simulink model "JX_Kinect"  (Simulink 7.7)
settings: Solver=ode45  StartTime=0.0  StopTime=inf  FixedStep=sample_time  RelTol=1e-3
InitFcn:
  | sample_time=0.01;
undefined symbols (not defined in the file or in its folder): gray
libraries: vrlib x4, simulink_extras x3, nid_lib x2, vipsnks x1, utility x1
(part 1 of 2)
settings Model: Creator=ttcl3  LastModifiedBy=Jx
settings SolverCC: MaxConsecutiveMinStep=auto
settings DebuggingCC: MultiTaskRateTransMsg=warning

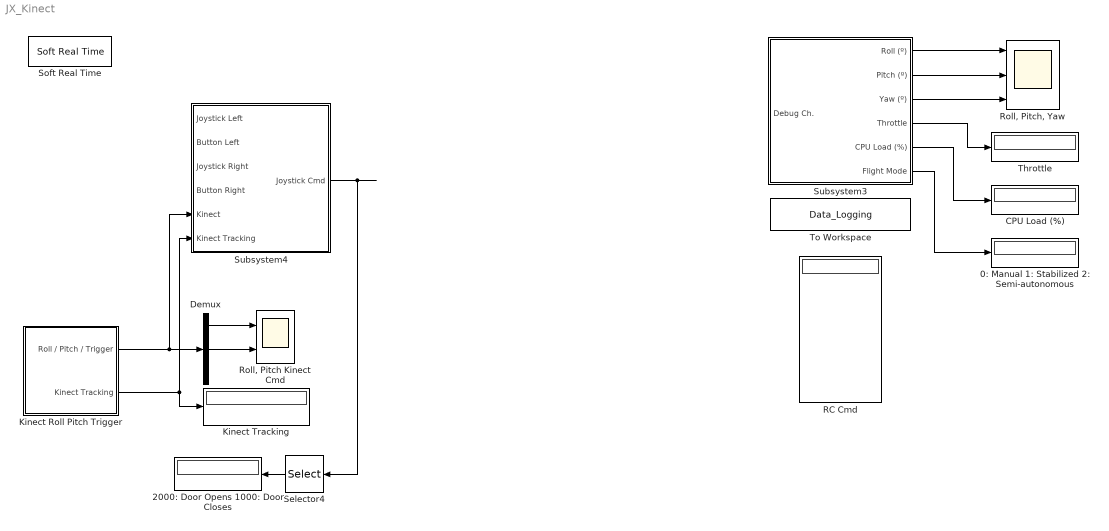
== system JX_Kinect ==
  0: Manual 1: Stabilized 2: Semi-autonomous : Display
  2000: Door Opens 1000: Door Closes : Display
  CPU Load (%) : Display
  Demux : Demux  Outputs=3
  Kinect Roll Pitch Trigger : Subsystem
      mask Display: image(imread('kinect.jpg'));port_label('output', 1, 'Roll/Pitch/Trigger'); port_label('output', 2, 'Tracking');
  Kinect Tracking : Display
  RC Cmd : Display
  "Roll, Pitch Kinect Cmd" : Scope  NumInputPorts=2
      settings: TickLabels=on  TimeRange=24  YMin=-90~-90  YMax=90~90  SampleInput=on
  "Roll, Pitch, Yaw" : Scope  NumInputPorts=3
      settings: TickLabels=on  TimeRange=24  YMin=-90~-90~-90  YMax=90~90~90  SampleInput=on
  Selector4 : Selector  InputPortWidth=7  IndexOptions=Index vector (dialog)  Indices=3  OutputSizes=1
  Soft Real Time : utility/Soft Real Time  x=0.8
  Subsystem3 : Subsystem
  Subsystem4 : Subsystem
  Throttle : Display
  To Workspace : ToWorkspace  VariableName=Data_Logging  SampleTime=-1  SaveFormat=Structure With Time
  wires:
  ? -> RC Cmd/1
  Subsystem3/1(Roll (º)) -> "Roll, Pitch, Yaw"/1
  Subsystem3/2(Pitch (º)) -> "Roll, Pitch, Yaw"/2
  Subsystem3/3(Yaw (º)) -> "Roll, Pitch, Yaw"/3
  Subsystem3/4(Throttle) -> Throttle/1
  Subsystem3/5(CPU Load (%)) -> CPU Load (%)/1
  Subsystem3/6(Flight Mode) -> 0: Manual 1: Stabilized 2: Semi-autonomous/1
  ? -> Subsystem3/1(Debug Ch.), To Workspace/1
  Subsystem4/1(Joystick Cmd) -> Selector4/1
  Kinect Roll Pitch Trigger/1(Roll / Pitch / Trigger) -> Subsystem4/5(Kinect), Demux/1
  Selector4/1 -> 2000: Door Opens 1000: Door Closes/1
  Kinect Roll Pitch Trigger/2(Kinect Tracking) -> Kinect Tracking/1, Subsystem4/6(Kinect Tracking)
  Demux/1 -> "Roll, Pitch Kinect Cmd"/1
  Demux/2 -> "Roll, Pitch Kinect Cmd"/2

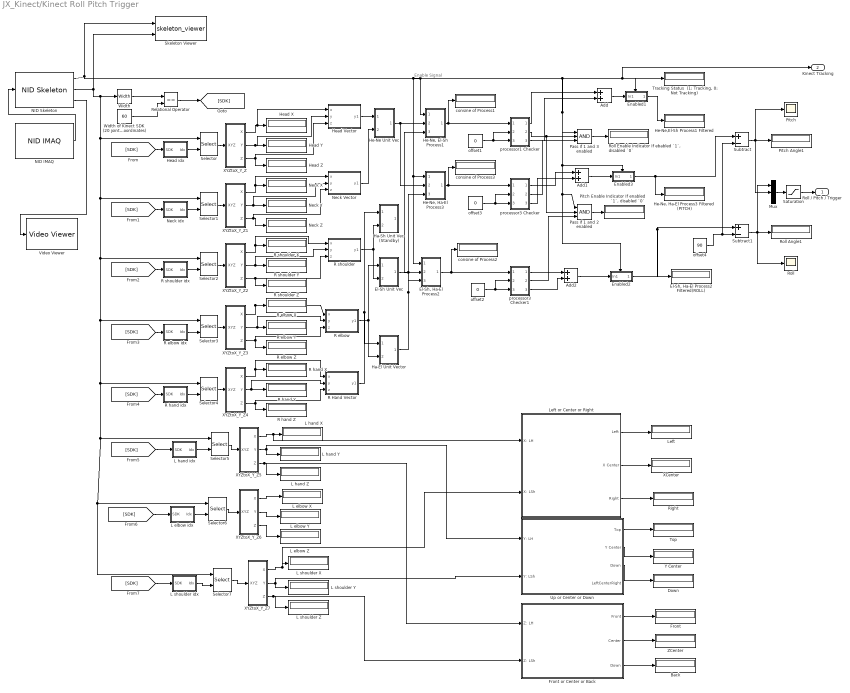
== system JX_Kinect/Kinect Roll Pitch Trigger ==
  note: Enable Signal
  Add : Sum
  Add1 : Sum
  Add2 : Sum
  Back : Display
  Down : Display
  El-Sh Unit Vec : Subsystem
  "El-Sh, Ha-El Process2" : Subsystem
  "El-Sh, Ha-El Process2 Filtered(ROLL)" : Display
  Enabled1 : Subsystem  TreatAsAtomicUnit=on
  Enabled2 : Subsystem  TreatAsAtomicUnit=on
  Enabled3 : Subsystem  TreatAsAtomicUnit=on
  Front : Display
  Front or Center or Back : Subsystem
  Ha-El Unit Vector : Subsystem
  Ha-Sh Unit Vec (Standby) : Subsystem
  He-Ne Unit Vec : Subsystem
  "He-Ne, El-Sh Process1" : Subsystem
  "He-Ne, Ha-El Process3" : Subsystem
  "He-Ne, Ha-El Process3 Filtered (PITCH)" : Display
  "He-Ne,El-Sh Process1 Filtered " : Display
  Head Vector : Stateflow chart  TreatAsAtomicUnit=on
  Head X : Display
  Head Y : Display
  Head Z : Display
  Head idx : Subsystem
  L elbow X : Display
  L elbow Y : Display
  L elbow Z : Display
  L elbow idx : Subsystem
  L hand X : Display
  L hand Y : Display
  L hand Z : Display
  L hand idx : Subsystem
  L shoulder X : Display
  L shoulder Y : Display
  L shoulder Z : Display
  L shoulder idx : Subsystem
  Left : Display
  Left or Center or Right : Subsystem
  Mux : Mux  Inputs=3
  NID IMAQ : nid_lib/NID IMAQ  imaq_depth=off  imaq_motion=off  imaq_image=off  view_point=off  imaq_skeleton=on  imaq_ir=off  mirror_image=off  imaq_sample_time=1/25  res_fps=VGA (640x480): 30 FPS  needPsiPose=off  angle_input=off  angle=0  angle_read=off  near_mode=off  seated_mode=off  skeleton_smooth=[1.0 0.5 0.5 0.05 0.04]  infer_skeleton=on
  NID Skeleton : nid_lib/NID Skeleton  num_of_skeleton_tracking=1  conv_XYZ_RW=on  viewer=on
  Neck Vector : Stateflow chart  TreatAsAtomicUnit=on
  Neck X : Display
  Neck Y : Display
  Neck Z : Display
  Neck idx : Subsystem
  Pass if 1 and 2 enabled : Logic  Inputs=3  AllPortsSameDT=off  OutDataTypeStr=boolean
  Pass if 1 and 3 enabled : Logic  Inputs=3  AllPortsSameDT=off  OutDataTypeStr=boolean
  Pitch : Scope
      settings: YMin=-90  YMax=90  SaveName=ScopeData3
  Pitch Angle1 : Display
  "Pitch Enable Indicator If enabled `1`, disabled `0` " : Display
  R Hand Vector : Stateflow chart  TreatAsAtomicUnit=on
  R elbow : Stateflow chart  TreatAsAtomicUnit=on
  R elbow X : Display
  R elbow Y : Display
  R elbow Z : Display
  R elbow idx : Subsystem
  R hand X : Display
  R hand Y : Display
  R hand Z : Display
  R hand idx : Subsystem
  R shoulder : Stateflow chart  TreatAsAtomicUnit=on
  R shoulder X : Display
  R shoulder Y : Display
  R shoulder Z : Display
  R shoulder idx : Subsystem
  Relational Operator : RelationalOperator  Operator===  OutDataTypeStr=boolean
  Right : Display
  Roll : Scope
      settings: YMin=-90  YMax=90  SaveName=ScopeData2
  Roll Angle1 : Display
  "Roll Enable Indicator If ebabled `1`, disabled `0`" : Display
  Saturation : Saturate  UpperLimit=30  LowerLimit=-30
  Selector{,1..7} (8 alike) : Selector  NumberOfDimensions=3  InputPortWidth=3  IndexOptions=Select all,Index vector (port),Select all  Indices=[1 3],1,1  OutputSizes=1,1,1
  Skeleton Viewer : M-S-Function  FunctionName=skeleton_viewer
      mask Display:
      | disp('Skeleton\nViewer')
      | 
      | port_label('input', 1, 'Tracking')
      | port_label('input', 2, 'Skeleton')
  Subtract : Sum  Inputs=+-
  Subtract1 : Sum  Inputs=+-
  Top : Display
  "Tracking Status  (1: Tracking, 0: Not Tracking)" : Display
  Up or Center or Down : Subsystem
  Video Viewer : vipsnks/Video Viewer  inputType=Obsolete7b  imagePorts=One multidimensional signal  useColorMap=off  colormapValue=gray(256)  specRange=off  minInputVal=0  maxInputVal=255  FigPos=[1181 519 698 403]  AxisZoom=on  trueSizedOnce=off  OpenAtMdlStart=on
  Width : Width
  Width of Kinect SDK  (20 joints x 3 coordinates) : Constant  Value=60
  XCenter : Display
  XYZtoX_Y_Z : Subsystem
  XYZtoX_Y_Z1 : Subsystem
  XYZtoX_Y_Z2 : Subsystem
  XYZtoX_Y_Z3 : Subsystem
  XYZtoX_Y_Z4 : Subsystem
  XYZtoX_Y_Z5 : Subsystem
  XYZtoX_Y_Z6 : Subsystem
  XYZtoX_Y_Z7 : Subsystem
  Y Center : Display
  ZCenter : Display
  consine of Process1 : Display
  consine of Process2 : Display
  consine of Process3 : Display
  offset1 : Constant  Value=0
  offset2 : Constant  Value=0
  offset3 : Constant  Value=0
  offset4 : Constant  Value=90
  processor1 Checker : Subsystem
  processor3 Checker : Subsystem
  processor3 Checker1 : Subsystem
  Roll / Pitch / Trigger : Outport
  Kinect Tracking : Outport  Port=2
  wires:
  Saturation/1 -> Roll / Pitch / Trigger/1
  Mux/1 -> Saturation/1
  Pass if 1 and 3 enabled/1 -> "Roll Enable Indicator If ebabled `1`, disabled `0`"/1
  Subtract1/1 -> Roll/1, Mux/1, Roll Angle1/1
  Subtract/1 -> Pitch/1, Mux/2, Pitch Angle1/1
  offset4/1 -> Subtract/2, Subtract1/2
  Add2/1 -> Enabled2/1(In1)
  processor3 Checker1/3(Out3) -> Add2/2
  processor3 Checker1/1(Out1) -> Add2/1
  processor3 Checker/3(Out3) -> Add1/2
  processor3 Checker/1(Out1) -> Add1/1
  Add1/1 -> Enabled3/1(In1)
  processor1 Checker/1(Out1) -> Add/1
  Add/1 -> Enabled1/1(In1)
  processor1 Checker/3(Out3) -> Add/2
  Enabled2/1(Out1) -> Subtract1/1, "El-Sh, Ha-El Process2 Filtered(ROLL)"/1
  Enabled1/1(Out1) -> "He-Ne,El-Sh Process1 Filtered "/1
  Enabled3/1(Out1) -> Subtract/1, "He-Ne, Ha-El Process3 Filtered (PITCH)"/1
  offset2/1 -> processor3 Checker1/2(In2), processor3 Checker1/3(In3)
  offset3/1 -> processor3 Checker/2(In2), processor3 Checker/3(In3)
  offset1/1 -> processor1 Checker/2(In2), processor1 Checker/3(In3)
  processor3 Checker1/2(Out2) -> Pass if 1 and 2 enabled/3
  processor1 Checker/2(Out2) -> Pass if 1 and 2 enabled/2, Pass if 1 and 3 enabled/2
  processor3 Checker/2(Out2) -> Pass if 1 and 3 enabled/3
  Pass if 1 and 2 enabled/1 -> "Pitch Enable Indicator If enabled `1`, disabled `0` "/1
  "El-Sh, Ha-El Process2"/1(Out1) -> processor3 Checker1/1(In1), consine of Process2/1
  "He-Ne, El-Sh Process1"/1(Out1) -> consine of Process1/1, processor1 Checker/1(In1)
  "He-Ne, Ha-El Process3"/1(Out1) -> processor3 Checker/1(In1), consine of Process3/1
  Ha-El Unit Vector/1(Out1) -> "He-Ne, Ha-El Process3"/3(In3), "El-Sh, Ha-El Process2"/3(In3)
  El-Sh Unit Vec/1(Out1) -> "El-Sh, Ha-El Process2"/2(In2), "He-Ne, El-Sh Process1"/3(In3)
  He-Ne Unit Vec/1(Out1) -> "He-Ne, El-Sh Process1"/2(In2), "He-Ne, Ha-El Process3"/2(In2)
  R elbow/1(y1) -> Ha-El Unit Vector/2(In2), El-Sh Unit Vec/1(In1)
  R Hand Vector/1(y1) -> Ha-El Unit Vector/1(In1), Ha-Sh Unit Vec (Standby)/1(In1)
  R shoulder/1(y1) -> El-Sh Unit Vec/2(In2), Ha-Sh Unit Vec (Standby)/2(In2)
  Head Vector/1(y1) -> He-Ne Unit Vec/1(In1)
  Neck Vector/1(y1) -> He-Ne Unit Vec/2(In2)
  Selector/1 -> XYZtoX_Y_Z/1(XYZ)
  Selector4/1 -> XYZtoX_Y_Z4/1(XYZ)
  XYZtoX_Y_Z4/3(Z) -> R Hand Vector/3(z), R hand Z/1
  XYZtoX_Y_Z4/2(Y) -> R Hand Vector/2(y), R hand Y/1
  XYZtoX_Y_Z4/1(X) -> R Hand Vector/1(x), R hand X/1
  Selector3/1 -> XYZtoX_Y_Z3/1(XYZ)
  XYZtoX_Y_Z3/3(Z) -> R elbow/3(z), R elbow Z/1
  XYZtoX_Y_Z3/2(Y) -> R elbow/2(y), R elbow Y/1
  XYZtoX_Y_Z3/1(X) -> R elbow/1(x), R elbow X/1
  Selector2/1 -> XYZtoX_Y_Z2/1(XYZ)
  XYZtoX_Y_Z2/3(Z) -> R shoulder/3(z), R shoulder Z/1
  XYZtoX_Y_Z2/2(Y) -> R shoulder/2(y), R shoulder Y/1
  XYZtoX_Y_Z2/1(X) -> R shoulder/1(x), R shoulder X/1
  XYZtoX_Y_Z1/3(Z) -> Neck Vector/3(z), Neck Z/1
  XYZtoX_Y_Z1/2(Y) -> Neck Vector/2(y), Neck Y/1
  XYZtoX_Y_Z1/1(X) -> Neck Vector/1(x), Neck X/1
  XYZtoX_Y_Z/3(Z) -> Head Vector/3(z), Head Z/1
  XYZtoX_Y_Z/2(Y) -> Head Vector/2(y), Head Y/1
  [SDK] -> R hand idx/1(SDK)
  R hand idx/1(Idx) -> Selector4/2
  [SDK] -> R elbow idx/1(SDK)
  R elbow idx/1(Idx) -> Selector3/2
  [SDK] -> R shoulder idx/1(SDK)
  R shoulder idx/1(Idx) -> Selector2/2
  Selector1/1 -> XYZtoX_Y_Z1/1(XYZ)
  [SDK] -> Neck idx/1(SDK)
  Neck idx/1(Idx) -> Selector1/2
  XYZtoX_Y_Z/1(X) -> Head Vector/1(x), Head X/1
  NID Skeleton/1 -> "He-Ne, El-Sh Process1"/1(In1), Pass if 1 and 3 enabled/1, Kinect Tracking/1, "Tracking Status  (1: Tracking, 0: Not Tracking)"/1, Enabled1/Enable, Enabled3/Enable, Enabled2/Enable, Pass if 1 and 2 enabled/1, "He-Ne, Ha-El Process3"/1(In1), "El-Sh, Ha-El Process2"/1(In1), Skeleton Viewer/1
  [SDK] -> Head idx/1(SDK)
  Head idx/1(Idx) -> Selector/2
  Relational Operator/1 -> [SDK]
  NID Skeleton/2 -> Selector3/1, Selector4/1, Selector5/1, Selector6/1, Selector7/1, Selector2/1, Selector1/1, Selector/1, Width/1, Skeleton Viewer/2
  Width of Kinect SDK  (20 joints x 3 coordinates)/1 -> Relational Operator/2
  Width/1 -> Relational Operator/1
  NID IMAQ/1 -> NID Skeleton/1
  [SDK] -> L hand idx/1(SDK)
  [SDK] -> L elbow idx/1(SDK)
  [SDK] -> L shoulder idx/1(SDK)
  L hand idx/1(Idx) -> Selector5/2
  L elbow idx/1(Idx) -> Selector6/2
  L shoulder idx/1(Idx) -> Selector7/2
  Selector5/1 -> XYZtoX_Y_Z5/1(XYZ)
  XYZtoX_Y_Z5/1(X) -> L hand X/1, Left or Center or Right/1(X: LH)
  XYZtoX_Y_Z5/2(Y) -> L hand Y/1, Up or Center or Down/1(Y: LH)
  XYZtoX_Y_Z5/3(Z) -> L hand Z/1, Front or Center or Back/1(Z: LH)
  XYZtoX_Y_Z6/1(X) -> L elbow X/1
  XYZtoX_Y_Z6/2(Y) -> L elbow Y/1
  XYZtoX_Y_Z6/3(Z) -> L elbow Z/1
  XYZtoX_Y_Z7/1(X) -> L shoulder X/1, Left or Center or Right/2(X: LSh)
  XYZtoX_Y_Z7/2(Y) -> L shoulder Y/1, Up or Center or Down/2(Y: LSh)
  XYZtoX_Y_Z7/3(Z) -> L shoulder Z/1, Front or Center or Back/2(Z: LSh)
  Selector6/1 -> XYZtoX_Y_Z6/1(XYZ)
  Selector7/1 -> XYZtoX_Y_Z7/1(XYZ)
  Left or Center or Right/1(Left) -> Left/1
  Left or Center or Right/3(Right) -> Right/1
  Up or Center or Down/1(Top) -> Top/1
  Up or Center or Down/2(Y Center) -> Y Center/1
  Up or Center or Down/3(Down) -> Down/1
  Front or Center or Back/1(Front) -> Front/1
  Front or Center or Back/2(Center) -> ZCenter/1
  Front or Center or Back/3(Down) -> Back/1
  Left or Center or Right/2(X Center) -> XCenter/1
  NID Skeleton/3 -> Video Viewer/1

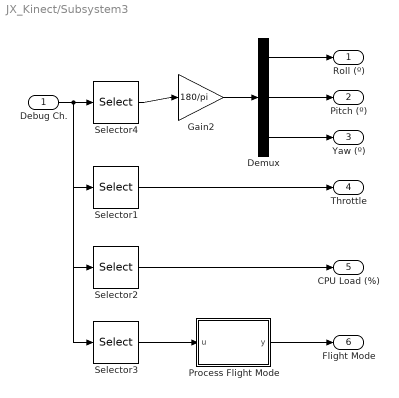
== system JX_Kinect/Subsystem3 ==
  Debug Ch. : Inport
  Demux : Demux  Outputs=3
  Gain2 : Gain  Gain=180/pi
  Process Flight Mode : Stateflow chart  TreatAsAtomicUnit=on
  Selector1 : Selector  InputPortWidth=6  IndexOptions=Index vector (dialog)  Indices=4  OutputSizes=1
  Selector2 : Selector  InputPortWidth=6  IndexOptions=Index vector (dialog)  Indices=5  OutputSizes=1
  Selector3 : Selector  InputPortWidth=6  IndexOptions=Index vector (dialog)  Indices=6  OutputSizes=1
  Selector4 : Selector  InputPortWidth=6  IndexOptions=Index vector (dialog)  Indices=[1 2 3]  OutputSizes=1
  Roll (º) : Outport
  Pitch (º) : Outport  Port=2
  Yaw (º) : Outport  Port=3
  Throttle : Outport  Port=4
  CPU Load (%) : Outport  Port=5
  Flight Mode : Outport  Port=6
  wires:
  Selector4/1 -> Gain2/1
  Gain2/1 -> Demux/1
  Demux/1 -> Roll (º)/1
  Demux/2 -> Pitch (º)/1
  Debug Ch./1 -> Selector4/1, Selector1/1, Selector2/1, Selector3/1
  Demux/3 -> Yaw (º)/1
  Selector1/1 -> Throttle/1
  Selector2/1 -> CPU Load (%)/1
  Selector3/1 -> Process Flight Mode/1(u)
  Process Flight Mode/1(y) -> Flight Mode/1

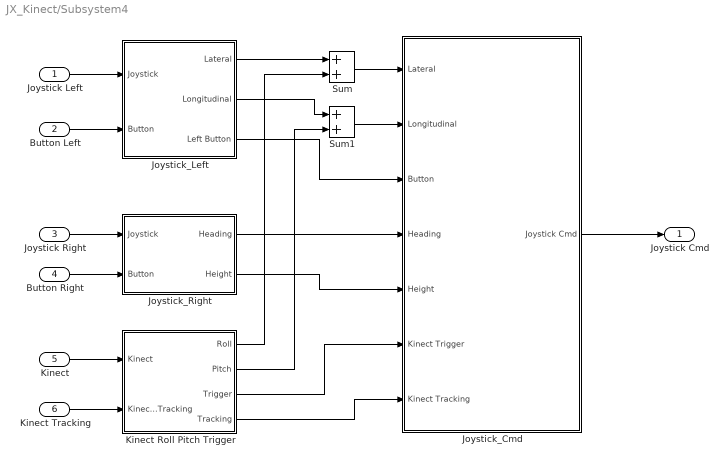
== system JX_Kinect/Subsystem4 ==
  Joystick Left : Inport
  Button Left : Inport  Port=2
  Joystick Right : Inport  Port=3
  Button Right : Inport  Port=4
  Kinect : Inport  Port=5
  Kinect Tracking : Inport  Port=6
  Joystick_Cmd : Subsystem
  Joystick_Left : Subsystem
  Joystick_Right : Subsystem
  Kinect Roll Pitch Trigger : Subsystem
  Sum : Sum
  Sum1 : Sum
  Joystick Cmd : Outport
  wires:
  Joystick Left/1 -> Joystick_Left/1(Joystick)
  Joystick Right/1 -> Joystick_Right/1(Joystick)
  Button Right/1 -> Joystick_Right/2(Button)
  Button Left/1 -> Joystick_Left/2(Button)
  Joystick_Right/1(Heading) -> Joystick_Cmd/4(Heading)
  Joystick_Right/2(Height) -> Joystick_Cmd/5(Height)
  Kinect/1 -> Kinect Roll Pitch Trigger/1(Kinect)
  Joystick_Left/3(Left Button) -> Joystick_Cmd/3(Button)
  Joystick_Cmd/1(Joystick Cmd) -> Joystick Cmd/1
  Joystick_Left/1(Lateral) -> Sum/1
  Sum/1 -> Joystick_Cmd/1(Lateral)
  Sum1/1 -> Joystick_Cmd/2(Longitudinal)
  Joystick_Left/2(Longitudinal) -> Sum1/1
  Kinect Roll Pitch Trigger/3(Trigger) -> Joystick_Cmd/6(Kinect Trigger)
  Kinect Tracking/1 -> Kinect Roll Pitch Trigger/2(Kinect Tracking)
  Kinect Roll Pitch Trigger/4(Tracking) -> Joystick_Cmd/7(Kinect Tracking)
  Kinect Roll Pitch Trigger/1(Roll) -> Sum/2
  Kinect Roll Pitch Trigger/2(Pitch) -> Sum1/2

== system JX_Kinect/Kinect Roll Pitch Trigger/El-Sh Unit Vec ==
  In1 : Inport
  In2 : Inport  Port=2
  Shoudler Elbow : vrlib/Utilities/Normalize Vector  SystemSampleTime=-1  maxzero=0
  Subtract3 : Sum  Inputs=+-
  Out1 : Outport
  wires:
  Shoudler Elbow/1 -> Out1/1
  In2/1 -> Subtract3/2
  In1/1 -> Subtract3/1
  Subtract3/1 -> Shoudler Elbow/1

== system JX_Kinect/Kinect Roll Pitch Trigger/El-Sh, Ha-El Process2 ==
  In1 : Inport
  In2 : Inport  Port=2
  In3 : Inport  Port=3
  Enabled Subsystem2 : Subsystem  TreatAsAtomicUnit=on
  "consine El-Sh, Ha-El" : DotProduct  InputSameDT=on  OutDataTypeStr=Inherit: Inherit via internal rule
  Out1 : Outport
  wires:
  Enabled Subsystem2/1(Out1) -> Out1/1
  In3/1 -> "consine El-Sh, Ha-El"/2
  In2/1 -> "consine El-Sh, Ha-El"/1
  In1/1 -> Enabled Subsystem2/Enable
  "consine El-Sh, Ha-El"/1 -> Enabled Subsystem2/1(In1)

== system JX_Kinect/Kinect Roll Pitch Trigger/Enabled1 ==
  In1 : Inport
  Enable : EnablePort
  Out1 : Outport
  wires:
  In1/1 -> Out1/1

== system JX_Kinect/Kinect Roll Pitch Trigger/Enabled2 ==
  In1 : Inport
  Enable : EnablePort
  Out1 : Outport
  wires:
  In1/1 -> Out1/1

== system JX_Kinect/Kinect Roll Pitch Trigger/Enabled3 ==
  In1 : Inport
  Enable : EnablePort
  Out1 : Outport
  wires:
  In1/1 -> Out1/1

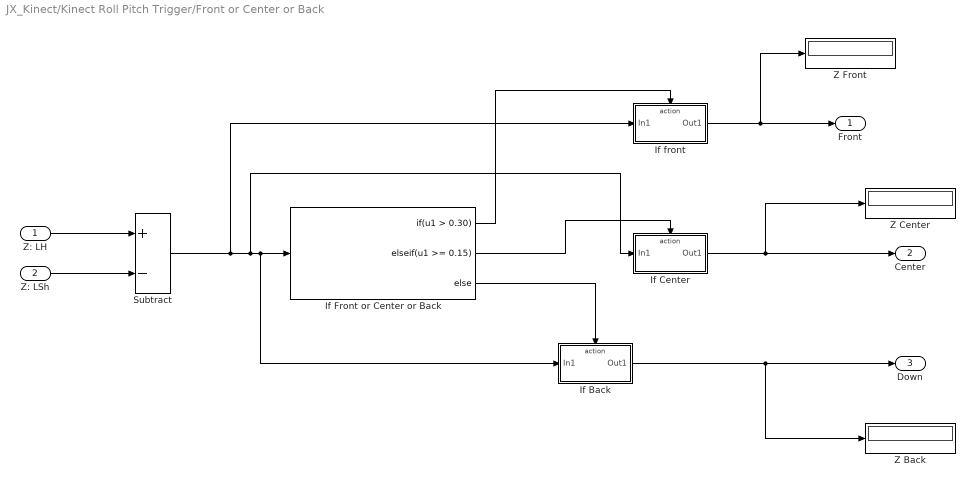
== system JX_Kinect/Kinect Roll Pitch Trigger/Front or Center or Back ==
  Z: LH : Inport
  Z: LSh : Inport  Port=2
  If Back : Subsystem  TreatAsAtomicUnit=on
  If Center : Subsystem  TreatAsAtomicUnit=on
  If Front or Center or Back : If  IfExpression=u1 > 0.30  ElseIfExpressions=u1 >= 0.15
  If front : Subsystem  TreatAsAtomicUnit=on
  Subtract : Sum  Inputs=+-
  Z Back : Display
  Z Center : Display
  Z Front : Display
  Front : Outport
  Center : Outport  Port=2
  Down : Outport  Port=3
  wires:
  Z: LH/1 -> Subtract/1
  Z: LSh/1 -> Subtract/2
  Subtract/1 -> If front/1(In1), If Center/1(In1), If Front or Center or Back/1, If Back/1(In1)
  If Front or Center or Back/1 -> If front/Action
  If front/1(Out1) -> Front/1, Z Front/1
  If Front or Center or Back/2 -> If Center/Action
  If Center/1(Out1) -> Center/1, Z Center/1
  If Front or Center or Back/3 -> If Back/Action
  If Back/1(Out1) -> Down/1, Z Back/1

== system JX_Kinect/Kinect Roll Pitch Trigger/Ha-El Unit Vector ==
  In1 : Inport
  In2 : Inport  Port=2
  Elbow Hand : vrlib/Utilities/Normalize Vector  SystemSampleTime=-1  maxzero=0
  Subtract2 : Sum  Inputs=+-
  Out1 : Outport
  wires:
  Elbow Hand/1 -> Out1/1
  In2/1 -> Subtract2/2
  In1/1 -> Subtract2/1
  Subtract2/1 -> Elbow Hand/1

== system JX_Kinect/Kinect Roll Pitch Trigger/Ha-Sh Unit Vec (Standby) ==
  In1 : Inport
  In2 : Inport  Port=2
  Subtract1 : Sum  Inputs=+-
  Unit Vector1 : vrlib/Utilities/Normalize Vector  SystemSampleTime=-1  maxzero=0
  Out1 : Outport
  wires:
  Unit Vector1/1 -> Out1/1
  In2/1 -> Subtract1/2
  In1/1 -> Subtract1/1
  Subtract1/1 -> Unit Vector1/1

== system JX_Kinect/Kinect Roll Pitch Trigger/He-Ne Unit Vec ==
  In1 : Inport
  In2 : Inport  Port=2
  Subtract : Sum  Inputs=+-
  Unit Vector : vrlib/Utilities/Normalize Vector  SystemSampleTime=-1  maxzero=0
  Out1 : Outport
  wires:
  In2/1 -> Subtract/2
  Unit Vector/1 -> Out1/1
  In1/1 -> Subtract/1
  Subtract/1 -> Unit Vector/1

== system JX_Kinect/Kinect Roll Pitch Trigger/He-Ne, El-Sh Process1 ==
  In1 : Inport
  In2 : Inport  Port=2
  In3 : Inport  Port=3
  Enabled Subsystem1 : Subsystem  TreatAsAtomicUnit=on
  consine He-Ne El-Sh : DotProduct  InputSameDT=on  OutDataTypeStr=Inherit: Inherit via internal rule
  Out1 : Outport
  wires:
  Enabled Subsystem1/1(Out1) -> Out1/1
  In3/1 -> consine He-Ne El-Sh/2
  In2/1 -> consine He-Ne El-Sh/1
  In1/1 -> Enabled Subsystem1/Enable
  consine He-Ne El-Sh/1 -> Enabled Subsystem1/1(In1)

== system JX_Kinect/Kinect Roll Pitch Trigger/He-Ne, Ha-El Process3 ==
  In1 : Inport
  In2 : Inport  Port=2
  In3 : Inport  Port=3
  Enabled Subsystem3 : Subsystem  TreatAsAtomicUnit=on
  "consine He-Ne, Ha-El" : DotProduct  InputSameDT=on  OutDataTypeStr=Inherit: Inherit via internal rule
  Out1 : Outport
  wires:
  Enabled Subsystem3/1(Out1) -> Out1/1
  In3/1 -> "consine He-Ne, Ha-El"/2
  In2/1 -> "consine He-Ne, Ha-El"/1
  In1/1 -> Enabled Subsystem3/Enable
  "consine He-Ne, Ha-El"/1 -> Enabled Subsystem3/1(In1)

== system JX_Kinect/Kinect Roll Pitch Trigger/Head idx ==
  SDK : Inport
  Kinect SDK : Constant  Value=4
  OpenNI : Constant
  Switch : Switch  Criteria=u2 ~= 0
  Idx : Outport
  wires:
  Switch/1 -> Idx/1
  SDK/1 -> Switch/2
  OpenNI/1 -> Switch/3
  Kinect SDK/1 -> Switch/1

== system JX_Kinect/Kinect Roll Pitch Trigger/L elbow idx ==
  SDK : Inport
  Kinect SDK : Constant  Value=6
  OpenNI : Constant  Value=8
  Switch : Switch  Criteria=u2 ~= 0
  Idx : Outport
  wires:
  Kinect SDK/1 -> Switch/1
  OpenNI/1 -> Switch/3
  SDK/1 -> Switch/2
  Switch/1 -> Idx/1

== system JX_Kinect/Kinect Roll Pitch Trigger/L hand idx ==
  SDK : Inport
  Kinect SDK : Constant  Value=8
  OpenNI : Constant  Value=9
  Switch : Switch  Criteria=u2 ~= 0
  Idx : Outport
  wires:
  Kinect SDK/1 -> Switch/1
  OpenNI/1 -> Switch/3
  SDK/1 -> Switch/2
  Switch/1 -> Idx/1

== system JX_Kinect/Kinect Roll Pitch Trigger/L shoulder idx ==
  SDK : Inport
  Kinect SDK : Constant  Value=5
  OpenNI : Constant  Value=7
  Switch : Switch  Criteria=u2 ~= 0
  Idx : Outport
  wires:
  Kinect SDK/1 -> Switch/1
  OpenNI/1 -> Switch/3
  SDK/1 -> Switch/2
  Switch/1 -> Idx/1

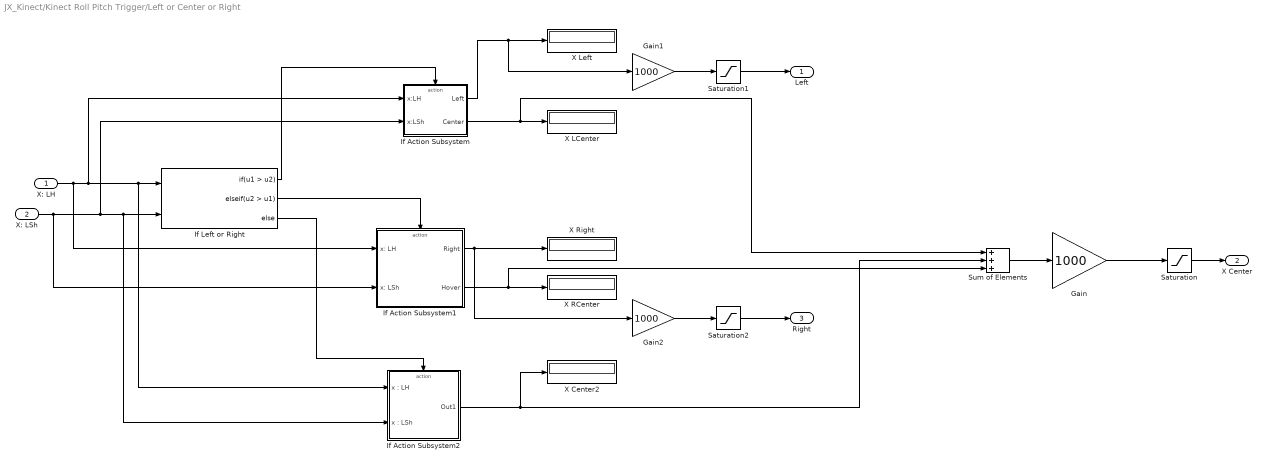
== system JX_Kinect/Kinect Roll Pitch Trigger/Left or Center or Right ==
  X: LH : Inport
  X: LSh : Inport  Port=2
  Gain : Gain  Gain=1000
  Gain1 : Gain  Gain=1000
  Gain2 : Gain  Gain=1000
  If Action Subsystem : Subsystem  TreatAsAtomicUnit=on
  If Action Subsystem1 : Subsystem  TreatAsAtomicUnit=on
  If Action Subsystem2 : Subsystem  TreatAsAtomicUnit=on
  If Left or Right : If  NumInputs=2  IfExpression=u1 > u2  ElseIfExpressions=u2 > u1
  Saturation : Saturate  UpperLimit=1  LowerLimit=0
  Saturation1 : Saturate  UpperLimit=1  LowerLimit=0
  Saturation2 : Saturate  UpperLimit=1  LowerLimit=0
  Sum of Elements : Sum  Inputs=+|+|+
  X Center2 : Display
  X LCenter : Display
  X Left : Display
  X RCenter : Display
  X Right : Display
  Left : Outport
  X Center : Outport  Port=2
  Right : Outport  Port=3
  wires:
  If Action Subsystem1/2(Hover) -> X RCenter/1, Sum of Elements/3
  If Action Subsystem1/1(Right) -> X Right/1, Gain2/1
  If Action Subsystem/2(Center) -> X LCenter/1, Sum of Elements/1
  If Left or Right/2 -> If Action Subsystem1/Action
  If Action Subsystem/1(Left) -> X Left/1, Gain1/1
  If Left or Right/1 -> If Action Subsystem/Action
  X: LH/1 -> If Action Subsystem/1(x:LH), If Left or Right/1, If Action Subsystem2/1("x : LH"), If Action Subsystem1/1(x: LH)
  X: LSh/1 -> If Action Subsystem/2(x:LSh), If Left or Right/2, If Action Subsystem2/2("x : LSh"), If Action Subsystem1/2(x: LSh)
  If Left or Right/3 -> If Action Subsystem2/Action
  If Action Subsystem2/1(Out1) -> X Center2/1, Sum of Elements/2
  Sum of Elements/1 -> Gain/1
  Gain/1 -> Saturation/1
  Saturation/1 -> X Center/1
  Gain1/1 -> Saturation1/1
  Saturation1/1 -> Left/1
  Gain2/1 -> Saturation2/1
  Saturation2/1 -> Right/1

== system JX_Kinect/Kinect Roll Pitch Trigger/Neck idx ==
  SDK : Inport
  Kinect SDK : Constant  Value=3
  OpenNI : Constant  Value=2
  Switch : Switch  Criteria=u2 ~= 0
  Idx : Outport
  wires:
  Kinect SDK/1 -> Switch/1
  OpenNI/1 -> Switch/3
  SDK/1 -> Switch/2
  Switch/1 -> Idx/1

== system JX_Kinect/Kinect Roll Pitch Trigger/R elbow idx ==
  SDK : Inport
  Kinect SDK : Constant  Value=10
  OpenNI : Constant  Value=5
  Switch : Switch  Criteria=u2 ~= 0
  Idx : Outport
  wires:
  Switch/1 -> Idx/1
  SDK/1 -> Switch/2
  OpenNI/1 -> Switch/3
  Kinect SDK/1 -> Switch/1

== system JX_Kinect/Kinect Roll Pitch Trigger/R hand idx ==
  SDK : Inport
  Kinect SDK : Constant  Value=12
  OpenNI : Constant  Value=6
  Switch : Switch  Criteria=u2 ~= 0
  Idx : Outport
  wires:
  Switch/1 -> Idx/1
  SDK/1 -> Switch/2
  OpenNI/1 -> Switch/3
  Kinect SDK/1 -> Switch/1

== system JX_Kinect/Kinect Roll Pitch Trigger/R shoulder idx ==
  SDK : Inport
  Kinect SDK : Constant  Value=9
  OpenNI : Constant  Value=4
  Switch : Switch  Criteria=u2 ~= 0
  Idx : Outport
  wires:
  Switch/1 -> Idx/1
  SDK/1 -> Switch/2
  OpenNI/1 -> Switch/3
  Kinect SDK/1 -> Switch/1

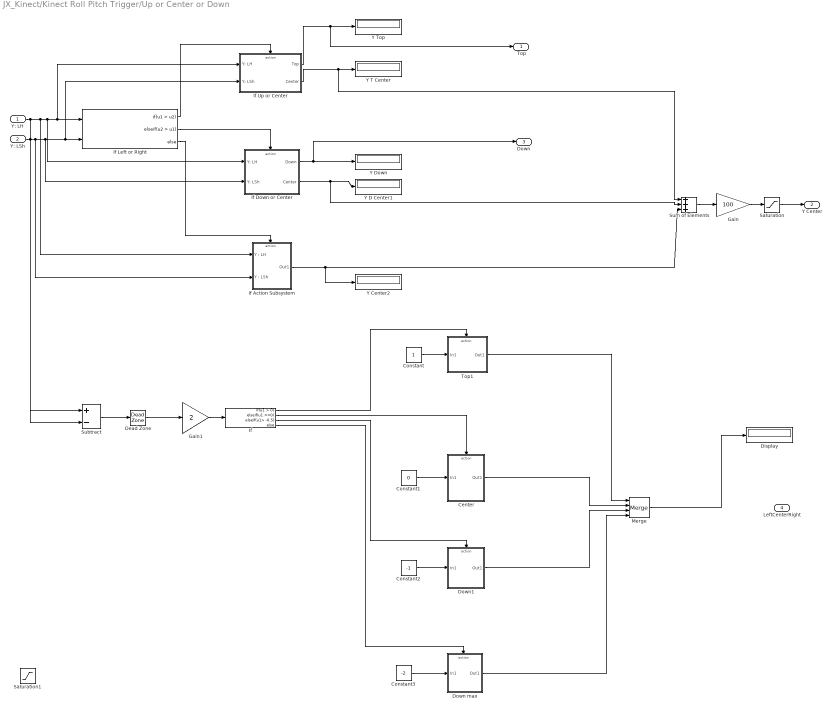
== system JX_Kinect/Kinect Roll Pitch Trigger/Up or Center or Down ==
  Y: LH : Inport
  Y: LSh : Inport  Port=2
  Center : Subsystem  TreatAsAtomicUnit=on
  Constant : Constant
  Constant1 : Constant  Value=0
  Constant2 : Constant  Value=-1
  Constant3 : Constant  Value=-2
  Dead Zone : DeadZone  LowerValue=-0.12  UpperValue=0.12  SaturateOnIntegerOverflow=on
  Display : Display
  Down max : Subsystem  TreatAsAtomicUnit=on
  Down1 : Subsystem  TreatAsAtomicUnit=on
  Gain : Gain  Gain=100
  Gain1 : Gain  Gain=2
  If : If  ElseIfExpressions=u1 ==0, u1> -0.5
  If Action Subsystem : Subsystem  TreatAsAtomicUnit=on
  If Down or Center : Subsystem  TreatAsAtomicUnit=on
  If Left or Right : If  NumInputs=2  IfExpression=u1 > u2  ElseIfExpressions=u2 > u1
  If Up or Center : Subsystem  TreatAsAtomicUnit=on
  Merge : Merge  Inputs=4
  Saturation : Saturate  UpperLimit=1  LowerLimit=0
  Saturation1 : Saturate  UpperLimit=1  LowerLimit=-1
  Subtract : Sum  Inputs=+-
  Sum of Elements : Sum  Inputs=+|+|+
  Top1 : Subsystem  TreatAsAtomicUnit=on
  Y Center2 : Display
  Y D Center1 : Display
  Y Down : Display
  Y T Center : Display
  Y Top : Display
  Top : Outport
  Y Center : Outport  Port=2
  Down : Outport  Port=3
  LeftCenterRight : Outport  Port=4
  wires:
  If Down or Center/2(Center) -> Y D Center1/1, Sum of Elements/2
  If Down or Center/1(Down) -> Y Down/1, Down/1
  If Up or Center/2(Center) -> Y T Center/1, Sum of Elements/1
  If Left or Right/2 -> If Down or Center/Action
  If Up or Center/1(Top) -> Y Top/1, Top/1
  If Left or Right/1 -> If Up or Center/Action
  Y: LH/1 -> If Left or Right/1, If Up or Center/1(Y: LH), If Down or Center/1(Y: LH), If Action Subsystem/1("Y : LH"), Subtract/1
  Y: LSh/1 -> If Left or Right/2, If Up or Center/2(Y: LSh), If Down or Center/2(Y: LSh), If Action Subsystem/2("Y : LSh"), Subtract/2
  If Left or Right/3 -> If Action Subsystem/Action
  If Action Subsystem/1(Out1) -> Y Center2/1, Sum of Elements/3
  Sum of Elements/1 -> Gain/1
  Gain/1 -> Saturation/1
  Saturation/1 -> Y Center/1
  Subtract/1 -> Dead Zone/1
  If/1 -> Top1/Action
  If/2 -> Center/Action
  If/3 -> Down1/Action
  If/4 -> Down max/Action
  Constant/1 -> Top1/1(In1)
  Dead Zone/1 -> Gain1/1
  Gain1/1 -> If/1
  Constant1/1 -> Center/1(In1)
  Constant2/1 -> Down1/1(In1)
  Constant3/1 -> Down max/1(In1)
  Center/1(Out1) -> Merge/2
  Down1/1(Out1) -> Merge/3
  Down max/1(Out1) -> Merge/4
  Top1/1(Out1) -> Merge/1
  Merge/1 -> Display/1

== system JX_Kinect/Kinect Roll Pitch Trigger/XYZtoX_Y_Z ==
  XYZ : Inport
  Selector : Selector  NumberOfDimensions=3  InputPortWidth=3  IndexOptions=Index vector (dialog),Index vector (dialog),Index vector (dialog)  Indices=1,1,1  OutputSizes=1,1,1
  Selector1 : Selector  NumberOfDimensions=3  InputPortWidth=3  IndexOptions=Index vector (dialog),Index vector (dialog),Index vector (dialog)  Indices=1,1,2  OutputSizes=1,1,1
  Selector2 : Selector  NumberOfDimensions=3  InputPortWidth=3  IndexOptions=Index vector (dialog),Index vector (dialog),Index vector (dialog)  Indices=1,1,3  OutputSizes=1,1,1
  X : Outport
  Y : Outport  Port=2
  Z : Outport  Port=3
  wires:
  Selector2/1 -> Z/1
  Selector1/1 -> Y/1
  Selector/1 -> X/1
  XYZ/1 -> Selector2/1, Selector1/1, Selector/1

== system JX_Kinect/Kinect Roll Pitch Trigger/XYZtoX_Y_Z1 ==
  XYZ : Inport
  Selector : Selector  NumberOfDimensions=3  InputPortWidth=3  IndexOptions=Index vector (dialog),Index vector (dialog),Index vector (dialog)  Indices=1,1,1  OutputSizes=1,1,1
  Selector1 : Selector  NumberOfDimensions=3  InputPortWidth=3  IndexOptions=Index vector (dialog),Index vector (dialog),Index vector (dialog)  Indices=1,1,2  OutputSizes=1,1,1
  Selector2 : Selector  NumberOfDimensions=3  InputPortWidth=3  IndexOptions=Index vector (dialog),Index vector (dialog),Index vector (dialog)  Indices=1,1,3  OutputSizes=1,1,1
  X : Outport
  Y : Outport  Port=2
  Z : Outport  Port=3
  wires:
  XYZ/1 -> Selector/1, Selector1/1, Selector2/1
  Selector/1 -> X/1
  Selector1/1 -> Y/1
  Selector2/1 -> Z/1

== system JX_Kinect/Kinect Roll Pitch Trigger/XYZtoX_Y_Z2 ==
  XYZ : Inport
  Selector : Selector  NumberOfDimensions=3  InputPortWidth=3  IndexOptions=Index vector (dialog),Index vector (dialog),Index vector (dialog)  Indices=1,1,1  OutputSizes=1,1,1
  Selector1 : Selector  NumberOfDimensions=3  InputPortWidth=3  IndexOptions=Index vector (dialog),Index vector (dialog),Index vector (dialog)  Indices=1,1,2  OutputSizes=1,1,1
  Selector2 : Selector  NumberOfDimensions=3  InputPortWidth=3  IndexOptions=Index vector (dialog),Index vector (dialog),Index vector (dialog)  Indices=1,1,3  OutputSizes=1,1,1
  X : Outport
  Y : Outport  Port=2
  Z : Outport  Port=3
  wires:
  Selector2/1 -> Z/1
  Selector1/1 -> Y/1
  Selector/1 -> X/1
  XYZ/1 -> Selector2/1, Selector1/1, Selector/1

== system JX_Kinect/Kinect Roll Pitch Trigger/XYZtoX_Y_Z3 ==
  XYZ : Inport
  Selector : Selector  NumberOfDimensions=3  InputPortWidth=3  IndexOptions=Index vector (dialog),Index vector (dialog),Index vector (dialog)  Indices=1,1,1  OutputSizes=1,1,1
  Selector1 : Selector  NumberOfDimensions=3  InputPortWidth=3  IndexOptions=Index vector (dialog),Index vector (dialog),Index vector (dialog)  Indices=1,1,2  OutputSizes=1,1,1
  Selector2 : Selector  NumberOfDimensions=3  InputPortWidth=3  IndexOptions=Index vector (dialog),Index vector (dialog),Index vector (dialog)  Indices=1,1,3  OutputSizes=1,1,1
  X : Outport
  Y : Outport  Port=2
  Z : Outport  Port=3
  wires:
  XYZ/1 -> Selector/1, Selector1/1, Selector2/1
  Selector/1 -> X/1
  Selector1/1 -> Y/1
  Selector2/1 -> Z/1

== system JX_Kinect/Kinect Roll Pitch Trigger/XYZtoX_Y_Z4 ==
  XYZ : Inport
  Selector : Selector  NumberOfDimensions=3  InputPortWidth=3  IndexOptions=Index vector (dialog),Index vector (dialog),Index vector (dialog)  Indices=1,1,1  OutputSizes=1,1,1
  Selector1 : Selector  NumberOfDimensions=3  InputPortWidth=3  IndexOptions=Index vector (dialog),Index vector (dialog),Index vector (dialog)  Indices=1,1,2  OutputSizes=1,1,1
  Selector2 : Selector  NumberOfDimensions=3  InputPortWidth=3  IndexOptions=Index vector (dialog),Index vector (dialog),Index vector (dialog)  Indices=1,1,3  OutputSizes=1,1,1
  X : Outport
  Y : Outport  Port=2
  Z : Outport  Port=3
  wires:
  Selector2/1 -> Z/1
  Selector1/1 -> Y/1
  Selector/1 -> X/1
  XYZ/1 -> Selector2/1, Selector1/1, Selector/1

== system JX_Kinect/Kinect Roll Pitch Trigger/XYZtoX_Y_Z5 ==
  XYZ : Inport
  Selector : Selector  NumberOfDimensions=3  InputPortWidth=3  IndexOptions=Index vector (dialog),Index vector (dialog),Index vector (dialog)  Indices=1,1,1  OutputSizes=1,1,1
  Selector1 : Selector  NumberOfDimensions=3  InputPortWidth=3  IndexOptions=Index vector (dialog),Index vector (dialog),Index vector (dialog)  Indices=1,1,2  OutputSizes=1,1,1
  Selector2 : Selector  NumberOfDimensions=3  InputPortWidth=3  IndexOptions=Index vector (dialog),Index vector (dialog),Index vector (dialog)  Indices=1,1,3  OutputSizes=1,1,1
  X : Outport
  Y : Outport  Port=2
  Z : Outport  Port=3
  wires:
  XYZ/1 -> Selector/1, Selector1/1, Selector2/1
  Selector/1 -> X/1
  Selector1/1 -> Y/1
  Selector2/1 -> Z/1

== system JX_Kinect/Kinect Roll Pitch Trigger/XYZtoX_Y_Z6 ==
  XYZ : Inport
  Selector : Selector  NumberOfDimensions=3  InputPortWidth=3  IndexOptions=Index vector (dialog),Index vector (dialog),Index vector (dialog)  Indices=1,1,1  OutputSizes=1,1,1
  Selector1 : Selector  NumberOfDimensions=3  InputPortWidth=3  IndexOptions=Index vector (dialog),Index vector (dialog),Index vector (dialog)  Indices=1,1,2  OutputSizes=1,1,1
  Selector2 : Selector  NumberOfDimensions=3  InputPortWidth=3  IndexOptions=Index vector (dialog),Index vector (dialog),Index vector (dialog)  Indices=1,1,3  OutputSizes=1,1,1
  X : Outport
  Y : Outport  Port=2
  Z : Outport  Port=3
  wires:
  XYZ/1 -> Selector/1, Selector1/1, Selector2/1
  Selector/1 -> X/1
  Selector1/1 -> Y/1
  Selector2/1 -> Z/1

== system JX_Kinect/Kinect Roll Pitch Trigger/XYZtoX_Y_Z7 ==
  XYZ : Inport
  Selector : Selector  NumberOfDimensions=3  InputPortWidth=3  IndexOptions=Index vector (dialog),Index vector (dialog),Index vector (dialog)  Indices=1,1,1  OutputSizes=1,1,1
  Selector1 : Selector  NumberOfDimensions=3  InputPortWidth=3  IndexOptions=Index vector (dialog),Index vector (dialog),Index vector (dialog)  Indices=1,1,2  OutputSizes=1,1,1
  Selector2 : Selector  NumberOfDimensions=3  InputPortWidth=3  IndexOptions=Index vector (dialog),Index vector (dialog),Index vector (dialog)  Indices=1,1,3  OutputSizes=1,1,1
  X : Outport
  Y : Outport  Port=2
  Z : Outport  Port=3
  wires:
  XYZ/1 -> Selector/1, Selector1/1, Selector2/1
  Selector/1 -> X/1
  Selector1/1 -> Y/1
  Selector2/1 -> Z/1

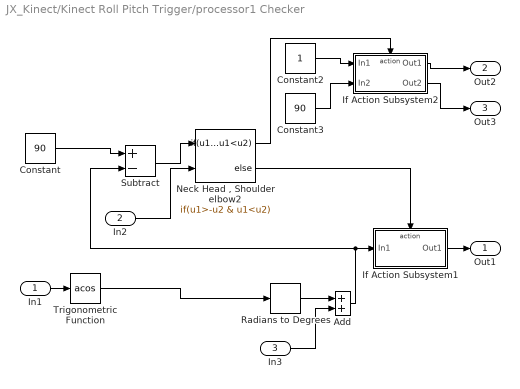
== system JX_Kinect/Kinect Roll Pitch Trigger/processor1 Checker ==
  In1 : Inport
  In2 : Inport  Port=2
  In3 : Inport  Port=3
  Add : Sum
  Constant : Constant  Value=90
  Constant2 : Constant
  Constant3 : Constant  Value=90
  If Action Subsystem1 : Subsystem  TreatAsAtomicUnit=on
  If Action Subsystem2 : Subsystem  TreatAsAtomicUnit=on
  "Neck Head , Shoulder elbow2" : If  NumInputs=2  IfExpression=u1>-u2 & u1<u2
  Radians to Degrees : simulink_extras/Transformations/Radians to Degrees  SystemSampleTime=-1
  Subtract : Sum  Inputs=+-
  Trigonometric Function : Trigonometry  Operator=acos
  Out1 : Outport
  Out2 : Outport  Port=2
  Out3 : Outport  Port=3
  wires:
  If Action Subsystem2/2(Out2) -> Out3/1
  Constant3/1 -> If Action Subsystem2/2(In2)
  Trigonometric Function/1 -> Radians to Degrees/1
  In3/1 -> Add/2
  Add/1 -> Subtract/2, If Action Subsystem1/1(In1)
  Radians to Degrees/1 -> Add/1
  Constant/1 -> Subtract/1
  "Neck Head , Shoulder elbow2"/1 -> If Action Subsystem2/Action
  If Action Subsystem2/1(Out1) -> Out2/1
  Constant2/1 -> If Action Subsystem2/1(In1)
  In1/1 -> Trigonometric Function/1
  If Action Subsystem1/1(Out1) -> Out1/1
  "Neck Head , Shoulder elbow2"/2 -> If Action Subsystem1/Action
  In2/1 -> "Neck Head , Shoulder elbow2"/2
  Subtract/1 -> "Neck Head , Shoulder elbow2"/1

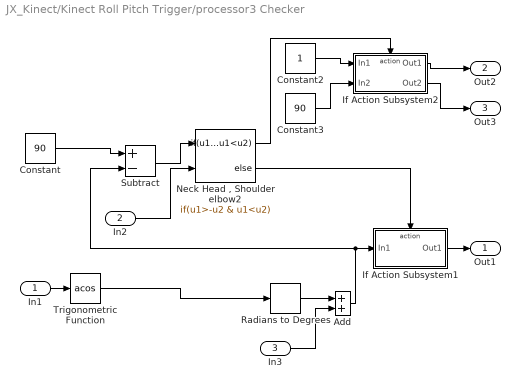
== system JX_Kinect/Kinect Roll Pitch Trigger/processor3 Checker ==
  In1 : Inport
  In2 : Inport  Port=2
  In3 : Inport  Port=3
  Add : Sum
  Constant : Constant  Value=90
  Constant2 : Constant
  Constant3 : Constant  Value=90
  If Action Subsystem1 : Subsystem  TreatAsAtomicUnit=on
  If Action Subsystem2 : Subsystem  TreatAsAtomicUnit=on
  "Neck Head , Shoulder elbow2" : If  NumInputs=2  IfExpression=u1>-u2 & u1<u2
  Radians to Degrees : simulink_extras/Transformations/Radians to Degrees  SystemSampleTime=-1
  Subtract : Sum  Inputs=+-
  Trigonometric Function : Trigonometry  Operator=acos
  Out1 : Outport
  Out2 : Outport  Port=2
  Out3 : Outport  Port=3
  wires:
  If Action Subsystem2/2(Out2) -> Out3/1
  Constant3/1 -> If Action Subsystem2/2(In2)
  Trigonometric Function/1 -> Radians to Degrees/1
  In3/1 -> Add/2
  Add/1 -> Subtract/2, If Action Subsystem1/1(In1)
  Radians to Degrees/1 -> Add/1
  Constant/1 -> Subtract/1
  "Neck Head , Shoulder elbow2"/1 -> If Action Subsystem2/Action
  If Action Subsystem2/1(Out1) -> Out2/1
  Constant2/1 -> If Action Subsystem2/1(In1)
  In1/1 -> Trigonometric Function/1
  If Action Subsystem1/1(Out1) -> Out1/1
  "Neck Head , Shoulder elbow2"/2 -> If Action Subsystem1/Action
  In2/1 -> "Neck Head , Shoulder elbow2"/2
  Subtract/1 -> "Neck Head , Shoulder elbow2"/1

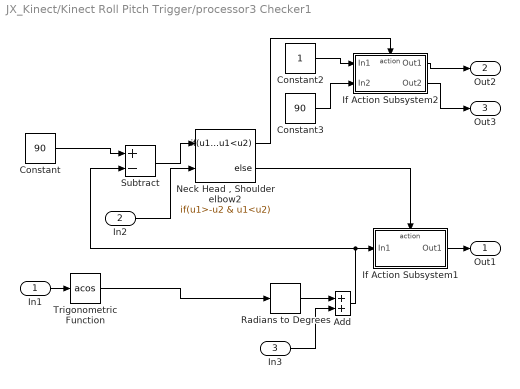
== system JX_Kinect/Kinect Roll Pitch Trigger/processor3 Checker1 ==
  In1 : Inport
  In2 : Inport  Port=2
  In3 : Inport  Port=3
  Add : Sum
  Constant : Constant  Value=90
  Constant2 : Constant
  Constant3 : Constant  Value=90
  If Action Subsystem1 : Subsystem  TreatAsAtomicUnit=on
  If Action Subsystem2 : Subsystem  TreatAsAtomicUnit=on
  "Neck Head , Shoulder elbow2" : If  NumInputs=2  IfExpression=u1>-u2 & u1<u2
  Radians to Degrees : simulink_extras/Transformations/Radians to Degrees  SystemSampleTime=-1
  Subtract : Sum  Inputs=+-
  Trigonometric Function : Trigonometry  Operator=acos
  Out1 : Outport
  Out2 : Outport  Port=2
  Out3 : Outport  Port=3
  wires:
  If Action Subsystem2/2(Out2) -> Out3/1
  Constant3/1 -> If Action Subsystem2/2(In2)
  Trigonometric Function/1 -> Radians to Degrees/1
  In3/1 -> Add/2
  Add/1 -> Subtract/2, If Action Subsystem1/1(In1)
  Radians to Degrees/1 -> Add/1
  Constant/1 -> Subtract/1
  "Neck Head , Shoulder elbow2"/1 -> If Action Subsystem2/Action
  If Action Subsystem2/1(Out1) -> Out2/1
  Constant2/1 -> If Action Subsystem2/1(In1)
  In1/1 -> Trigonometric Function/1
  If Action Subsystem1/1(Out1) -> Out1/1
  "Neck Head , Shoulder elbow2"/2 -> If Action Subsystem1/Action
  In2/1 -> "Neck Head , Shoulder elbow2"/2
  Subtract/1 -> "Neck Head , Shoulder elbow2"/1

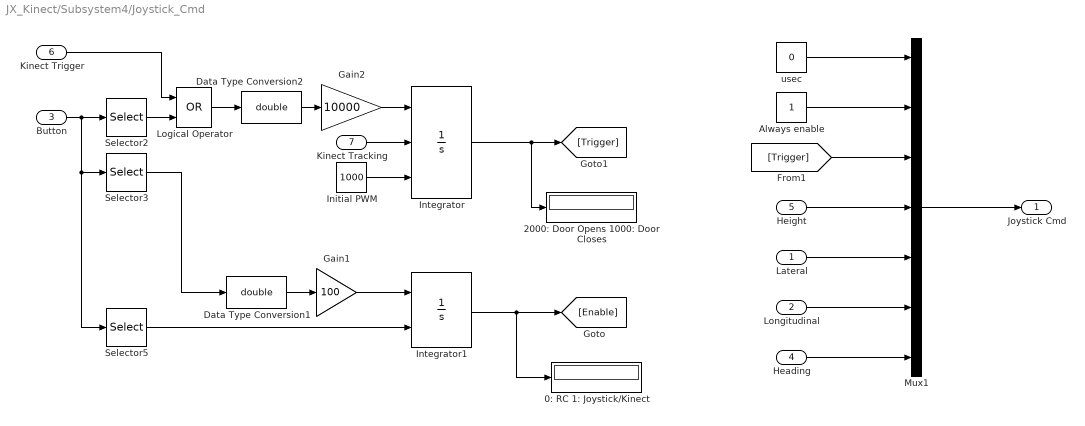
== system JX_Kinect/Subsystem4/Joystick_Cmd ==
  Lateral : Inport
  Longitudinal : Inport  Port=2
  Button : Inport  Port=3
  Heading : Inport  Port=4
  Height : Inport  Port=5
  Kinect Trigger : Inport  Port=6
  Kinect Tracking : Inport  Port=7
  0: RC 1: Joystick/Kinect : Display
  2000: Door Opens 1000: Door Closes : Display
  Always enable : Constant  SampleTime=sample_time
  Data Type Conversion1 : DataTypeConversion  OutDataTypeStr=double
  Data Type Conversion2 : DataTypeConversion  OutDataTypeStr=double
  Gain1 : Gain  Gain=100
  Gain2 : Gain  Gain=10000
  Initial PWM : Constant  Value=1000
  Integrator : Integrator  ExternalReset=falling  InitialConditionSource=external  LimitOutput=on  UpperSaturationLimit=2000  LowerSaturationLimit=1000
  Integrator1 : Integrator  ExternalReset=either  LimitOutput=on  UpperSaturationLimit=1  LowerSaturationLimit=0
  Logical Operator : Logic  Operator=OR  AllPortsSameDT=off  OutDataTypeStr=boolean
  Mux1 : Mux  Inputs=7
  Selector2 : Selector  InputPortWidth=12  IndexOptions=Index vector (dialog)  Indices=1  OutputSizes=1
  Selector3 : Selector  InputPortWidth=12  IndexOptions=Index vector (dialog)  Indices=4  OutputSizes=1
  Selector5 : Selector  InputPortWidth=12  IndexOptions=Index vector (dialog)  Indices=3  OutputSizes=1
  usec : Constant  Value=0  SampleTime=sample_time
  Joystick Cmd : Outport
  wires:
  usec/1 -> Mux1/1
  Mux1/1 -> Joystick Cmd/1
  Height/1 -> Mux1/4
  Lateral/1 -> Mux1/5
  Longitudinal/1 -> Mux1/6
  Heading/1 -> Mux1/7
  Button/1 -> Selector2/1, Selector5/1, Selector3/1
  Initial PWM/1 -> Integrator/3
  Selector3/1 -> Data Type Conversion1/1
  Data Type Conversion1/1 -> Gain1/1
  Gain1/1 -> Integrator1/1
  Selector5/1 -> Integrator1/2
  [Trigger] -> Mux1/3
  Integrator/1 -> 2000: Door Opens 1000: Door Closes/1, [Trigger]
  Integrator1/1 -> [Enable], 0: RC 1: Joystick/Kinect/1
  Selector2/1 -> Logical Operator/2
  Kinect Trigger/1 -> Logical Operator/1
  Data Type Conversion2/1 -> Gain2/1
  Logical Operator/1 -> Data Type Conversion2/1
  Gain2/1 -> Integrator/1
  Always enable/1 -> Mux1/2
  Kinect Tracking/1 -> Integrator/2

== system JX_Kinect/Subsystem4/Joystick_Left ==
  Joystick : Inport
  Button : Inport  Port=2
  Dead Zone : DeadZone  LowerValue=-0.1  UpperValue=0.1  SaturateOnIntegerOverflow=on
  Pitch Trim : Constant  Value=-0.018
  Roll Trim : Constant  Value=-0.017
  Selector1 : Selector  InputPortWidth=4  IndexOptions=Index vector (dialog)  Indices=2  OutputSizes=1
  Selector4 : Selector  InputPortWidth=4  IndexOptions=Index vector (dialog)  Indices=1  OutputSizes=1
  Sum : Sum
  Sum1 : Sum
  Lateral : Outport
  Longitudinal : Outport  Port=2
  Left Button : Outport  Port=3
  wires:
  Joystick/1 -> Dead Zone/1
  Roll Trim/1 -> Sum/2
  Pitch Trim/1 -> Sum1/2
  Dead Zone/1 -> Selector4/1, Selector1/1
  Selector4/1 -> Sum/1
  Selector1/1 -> Sum1/1
  Sum/1 -> Lateral/1
  Sum1/1 -> Longitudinal/1
  Button/1 -> Left Button/1

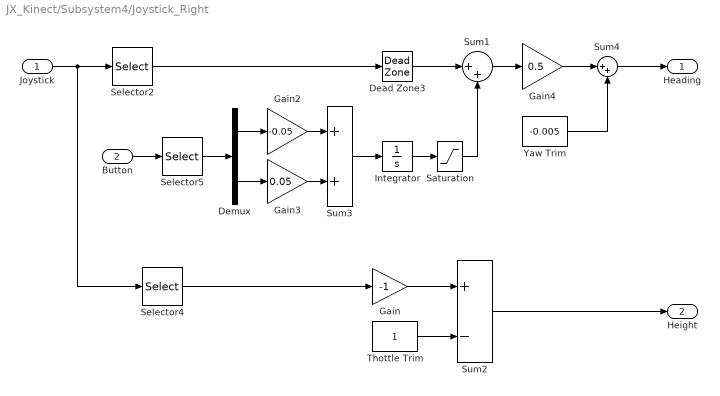
== system JX_Kinect/Subsystem4/Joystick_Right ==
  Joystick : Inport
  Button : Inport  Port=2
  Dead Zone3 : DeadZone  LowerValue=-0.2  UpperValue=0.2  SaturateOnIntegerOverflow=on
  Demux : Demux  Outputs=2
  Gain : Gain  Gain=-1
  Gain2 : Gain  Gain=-0.05
  Gain3 : Gain  Gain=0.05
  Gain4 : Gain  Gain=0.5
  Integrator : Integrator
  Saturation : Saturate  UpperLimit=0.1  LowerLimit=-0.1
  Selector2 : Selector  InputPortWidth=3  IndexOptions=Index vector (dialog)  Indices=[1]  OutputSizes=1
  Selector4 : Selector  InputPortWidth=3  IndexOptions=Index vector (dialog)  Indices=2  OutputSizes=1
  Selector5 : Selector  InputPortWidth=11  IndexOptions=Index vector (dialog)  Indices=[4 5]  OutputSizes=1
  Sum1 : Sum  Inputs=|++
  Sum2 : Sum  Inputs=+-
  Sum3 : Sum  OutDataTypeStr=double
  Sum4 : Sum  Inputs=|++
  Thottle Trim : Constant
  Yaw Trim : Constant  Value=-0.005
  Heading : Outport
  Height : Outport  Port=2
  wires:
  Selector2/1 -> Dead Zone3/1
  Selector4/1 -> Gain/1
  Joystick/1 -> Selector2/1, Selector4/1
  Gain/1 -> Sum2/1
  Thottle Trim/1 -> Sum2/2
  Sum2/1 -> Height/1
  Button/1 -> Selector5/1
  Selector5/1 -> Demux/1
  Demux/2 -> Gain3/1
  Demux/1 -> Gain2/1
  Gain2/1 -> Sum3/1
  Gain3/1 -> Sum3/2
  Sum3/1 -> Integrator/1
  Dead Zone3/1 -> Sum1/1
  Integrator/1 -> Saturation/1
  Saturation/1 -> Sum1/2
  Gain4/1 -> Sum4/1
  Yaw Trim/1 -> Sum4/2
  Sum4/1 -> Heading/1
  Sum1/1 -> Gain4/1

== system JX_Kinect/Subsystem4/Kinect Roll Pitch Trigger ==
  Kinect : Inport
  Kinect Tracking : Inport  Port=2
  Data Type Conversion : DataTypeConversion  OutDataTypeStr=boolean
  Demux : Demux  Outputs=3
  Scale sensitivity by one third1 : Gain  Gain=1/180
  Scale sensitivity by one third2 : Gain  Gain=1/180
  Scope1 : Scope
      settings: SaveName=ScopeData4
  Roll : Outport
  Pitch : Outport  Port=2
  Trigger : Outport  Port=3
  Tracking : Outport  Port=4
  wires:
  Kinect/1 -> Demux/1
  Demux/1 -> Scale sensitivity by one third1/1
  Demux/2 -> Scale sensitivity by one third2/1
  Demux/3 -> Trigger/1
  Scale sensitivity by one third1/1 -> Roll/1, Scope1/1
  Scale sensitivity by one third2/1 -> Pitch/1
  Kinect Tracking/1 -> Data Type Conversion/1
  Data Type Conversion/1 -> Tracking/1

== system JX_Kinect/Kinect Roll Pitch Trigger/El-Sh, Ha-El Process2/Enabled Subsystem2 ==
  In1 : Inport
  Enable : EnablePort
  Out1 : Outport
  wires:
  In1/1 -> Out1/1

== system JX_Kinect/Kinect Roll Pitch Trigger/Front or Center or Back/If Back ==
  In1 : Inport
  Action Port : ActionPort  ActionType=else
  Out1 : Outport
  wires:
  In1/1 -> Out1/1

== system JX_Kinect/Kinect Roll Pitch Trigger/Front or Center or Back/If Center ==
  In1 : Inport
  Action Port : ActionPort  ActionType=elseif
  Out1 : Outport
  wires:
  In1/1 -> Out1/1

== system JX_Kinect/Kinect Roll Pitch Trigger/Front or Center or Back/If front ==
  In1 : Inport
  Action Port : ActionPort  ActionType=then
  Out1 : Outport
  wires:
  In1/1 -> Out1/1

== system JX_Kinect/Kinect Roll Pitch Trigger/He-Ne, El-Sh Process1/Enabled Subsystem1 ==
  In1 : Inport
  Enable : EnablePort
  Out1 : Outport
  wires:
  In1/1 -> Out1/1

== system JX_Kinect/Kinect Roll Pitch Trigger/He-Ne, Ha-El Process3/Enabled Subsystem3 ==
  In1 : Inport
  Enable : EnablePort
  Out1 : Outport
  wires:
  In1/1 -> Out1/1

== system JX_Kinect/Kinect Roll Pitch Trigger/Left or Center or Right/If Action Subsystem ==
  x:LH : Inport
  x:LSh : Inport  Port=2
  Action Port : ActionPort  ActionType=then
  Buffer : Constant  Value=0.14
  Display : Display
  Display1 : Display
  Else Center : Subsystem  TreatAsAtomicUnit=on
  If : If
  If Left : Subsystem  TreatAsAtomicUnit=on
  Subtract1 : Sum  Inputs=+-
  Subtract2 : Sum  Inputs=+-
  Left : Outport
  Center : Outport  Port=2
  wires:
  Buffer/1 -> Subtract2/2
  Subtract2/1 -> If/1, If Left/1(In1), Else Center/1(In1)
  If/1 -> If Left/Action
  If Left/1(Out1) -> Left/1, Display1/1
  Else Center/1(Out1) -> Center/1, Display/1
  x:LH/1 -> Subtract1/1
  x:LSh/1 -> Subtract1/2
  If/2 -> Else Center/Action
  Subtract1/1 -> Subtract2/1

== system JX_Kinect/Kinect Roll Pitch Trigger/Left or Center or Right/If Action Subsystem1 ==
  x: LH : Inport
  x: LSh : Inport  Port=2
  Action Port : ActionPort  ActionType=elseif
  Buffer : Constant  Value=0.14
  Else Hover : Subsystem  TreatAsAtomicUnit=on
  If : If
  If Right : Subsystem  TreatAsAtomicUnit=on
  Subtract1 : Sum  Inputs=+-
  Subtract2 : Sum  Inputs=+-
  Right : Outport
  Hover : Outport  Port=2
  wires:
  Buffer/1 -> Subtract2/2
  Subtract2/1 -> If/1, If Right/1(In1), Else Hover/1(In1)
  If/1 -> If Right/Action
  If Right/1(Out1) -> Right/1
  If/2 -> Else Hover/Action
  Else Hover/1(Out1) -> Hover/1
  x: LSh/1 -> Subtract1/1
  x: LH/1 -> Subtract1/2
  Subtract1/1 -> Subtract2/1

== system JX_Kinect/Kinect Roll Pitch Trigger/Left or Center or Right/If Action Subsystem2 ==
  "x : LH" : Inport
  "x : LSh" : Inport  Port=2
  Action Port : ActionPort  ActionType=else
  Subtract : Sum  Inputs=+-
  Out1 : Outport
  wires:
  "x : LH"/1 -> Subtract/1
  "x : LSh"/1 -> Subtract/2
  Subtract/1 -> Out1/1

== system JX_Kinect/Kinect Roll Pitch Trigger/Up or Center or Down/Center ==
  In1 : Inport
  Action Port : ActionPort  ActionType=elseif
  Out1 : Outport
  wires:
  In1/1 -> Out1/1

== system JX_Kinect/Kinect Roll Pitch Trigger/Up or Center or Down/Down max ==
  In1 : Inport
  Action Port : ActionPort  ActionType=else
  Out1 : Outport
  wires:
  In1/1 -> Out1/1

== system JX_Kinect/Kinect Roll Pitch Trigger/Up or Center or Down/Down1 ==
  In1 : Inport
  Action Port : ActionPort  ActionType=elseif
  Out1 : Outport
  wires:
  In1/1 -> Out1/1

== system JX_Kinect/Kinect Roll Pitch Trigger/Up or Center or Down/If Action Subsystem ==
  "Y : LH" : Inport
  "Y : LSh" : Inport  Port=2
  Action Port : ActionPort  ActionType=else
  Subtract : Sum  Inputs=+-
  Out1 : Outport
  wires:
  "Y : LH"/1 -> Subtract/1
  "Y : LSh"/1 -> Subtract/2
  Subtract/1 -> Out1/1

== system JX_Kinect/Kinect Roll Pitch Trigger/Up or Center or Down/If Down or Center ==
  Y: LH : Inport
  Y: LSh : Inport  Port=2
  Action Port : ActionPort  ActionType=elseif
  Buffer : Constant  Value=0.14
  Else Center : Subsystem  TreatAsAtomicUnit=on
  If : If
  If Down : Subsystem  TreatAsAtomicUnit=on
  Subtract1 : Sum  Inputs=+-
  Subtract2 : Sum  Inputs=+-
  Down : Outport
  Center : Outport  Port=2
  wires:
  Buffer/1 -> Subtract2/2
  Subtract2/1 -> If/1, If Down/1(In1), Else Center/1(In1)
  If/1 -> If Down/Action
  If Down/1(Out1) -> Down/1
  If/2 -> Else Center/Action
  Else Center/1(Out1) -> Center/1
  Y: LSh/1 -> Subtract1/1
  Y: LH/1 -> Subtract1/2
  Subtract1/1 -> Subtract2/1

== system JX_Kinect/Kinect Roll Pitch Trigger/Up or Center or Down/If Up or Center ==
  Y: LH : Inport
  Y: LSh : Inport  Port=2
  Action Port : ActionPort  ActionType=then
  Buffer : Constant  Value=0.23
  Else Center : Subsystem  TreatAsAtomicUnit=on
  If : If
  If Top : Subsystem  TreatAsAtomicUnit=on
  Subtract1 : Sum  Inputs=+-
  Subtract2 : Sum  Inputs=+-
  Top : Outport
  Center : Outport  Port=2
  wires:
  Buffer/1 -> Subtract2/2
  Subtract2/1 -> If/1, If Top/1(In1), Else Center/1(In1)
  If/1 -> If Top/Action
  If Top/1(Out1) -> Top/1
  If/2 -> Else Center/Action
  Else Center/1(Out1) -> Center/1
  Y: LH/1 -> Subtract1/1
  Y: LSh/1 -> Subtract1/2
  Subtract1/1 -> Subtract2/1

== system JX_Kinect/Kinect Roll Pitch Trigger/Up or Center or Down/Top1 ==
  In1 : Inport
  Action Port : ActionPort  ActionType=then
  Out1 : Outport
  wires:
  In1/1 -> Out1/1

== system JX_Kinect/Kinect Roll Pitch Trigger/processor1 Checker/If Action Subsystem1 ==
  In1 : Inport
  Action Port : ActionPort  ActionType=else
  Out1 : Outport  OutputWhenDisabled=reset  InitialOutput=[0.00000]
  wires:
  In1/1 -> Out1/1

== system JX_Kinect/Kinect Roll Pitch Trigger/processor1 Checker/If Action Subsystem2 ==
  In1 : Inport
  In2 : Inport  Port=2
  Action Port : ActionPort  ActionType=then
  Out1 : Outport  OutputWhenDisabled=reset  InitialOutput=[0]
  Out2 : Outport  Port=2  OutputWhenDisabled=reset  InitialOutput=[0]
  wires:
  In2/1 -> Out2/1
  In1/1 -> Out1/1

== system JX_Kinect/Kinect Roll Pitch Trigger/processor3 Checker/If Action Subsystem1 ==
  In1 : Inport
  Action Port : ActionPort  ActionType=else
  Out1 : Outport  OutputWhenDisabled=reset  InitialOutput=[0.00000]
  wires:
  In1/1 -> Out1/1

== system JX_Kinect/Kinect Roll Pitch Trigger/processor3 Checker/If Action Subsystem2 ==
  In1 : Inport
  In2 : Inport  Port=2
  Action Port : ActionPort  ActionType=then
  Out1 : Outport  OutputWhenDisabled=reset  InitialOutput=[0]
  Out2 : Outport  Port=2  OutputWhenDisabled=reset  InitialOutput=[0]
  wires:
  In2/1 -> Out2/1
  In1/1 -> Out1/1

== system JX_Kinect/Kinect Roll Pitch Trigger/processor3 Checker1/If Action Subsystem1 ==
  In1 : Inport
  Action Port : ActionPort  ActionType=else
  Out1 : Outport  OutputWhenDisabled=reset  InitialOutput=[0.00000]
  wires:
  In1/1 -> Out1/1

== system JX_Kinect/Kinect Roll Pitch Trigger/processor3 Checker1/If Action Subsystem2 ==
  In1 : Inport
  In2 : Inport  Port=2
  Action Port : ActionPort  ActionType=then
  Out1 : Outport  OutputWhenDisabled=reset  InitialOutput=[0]
  Out2 : Outport  Port=2  OutputWhenDisabled=reset  InitialOutput=[0]
  wires:
  In2/1 -> Out2/1
  In1/1 -> Out1/1

== system JX_Kinect/Kinect Roll Pitch Trigger/Left or Center or Right/If Action Subsystem/Else Center ==
  In1 : Inport
  Action Port : ActionPort  InitializeStates=reset  ActionType=else
  Abs : Abs
  Out1 : Outport
  wires:
  In1/1 -> Abs/1
  Abs/1 -> Out1/1

== system JX_Kinect/Kinect Roll Pitch Trigger/Left or Center or Right/If Action Subsystem/If Left ==
  In1 : Inport
  Action Port : ActionPort  InitializeStates=reset  ActionType=then
  Out1 : Outport
  wires:
  In1/1 -> Out1/1

== system JX_Kinect/Kinect Roll Pitch Trigger/Left or Center or Right/If Action Subsystem1/Else Hover ==
  In1 : Inport
  Action Port : ActionPort  ActionType=else
  Abs : Abs
  Out1 : Outport
  wires:
  In1/1 -> Abs/1
  Abs/1 -> Out1/1

== system JX_Kinect/Kinect Roll Pitch Trigger/Left or Center or Right/If Action Subsystem1/If Right ==
  In1 : Inport
  Action Port : ActionPort  ActionType=then
  Out1 : Outport
  wires:
  In1/1 -> Out1/1

== system JX_Kinect/Kinect Roll Pitch Trigger/Up or Center or Down/If Down or Center/Else Center ==
  In1 : Inport
  Action Port : ActionPort  ActionType=else
  Abs : Abs
  Out1 : Outport
  wires:
  In1/1 -> Abs/1
  Abs/1 -> Out1/1

== system JX_Kinect/Kinect Roll Pitch Trigger/Up or Center or Down/If Down or Center/If Down ==
  In1 : Inport
  Action Port : ActionPort  ActionType=then
  Out1 : Outport
  wires:
  In1/1 -> Out1/1

== system JX_Kinect/Kinect Roll Pitch Trigger/Up or Center or Down/If Up or Center/Else Center ==
  In1 : Inport
  Action Port : ActionPort  ActionType=else
  Abs : Abs
  Out1 : Outport
  wires:
  In1/1 -> Abs/1
  Abs/1 -> Out1/1

== system JX_Kinect/Kinect Roll Pitch Trigger/Up or Center or Down/If Up or Center/If Top ==
  In1 : Inport
  Action Port : ActionPort  ActionType=then
  Out1 : Outport
  wires:
  In1/1 -> Out1/1

== matlab function Kinect Roll Pitch Trigger/Head Vector ==
  data: x input double; y input double; z input double; y1 output double
function y1 = fcn(x,y,z)
%#codegen
y1 = [x,y,z];

== matlab function Subsystem3/Process Flight Mode ==
  data: u input double; y output double
function y = fcn(u)
%#codegen

if u <=-0.5
    y = 0;  % Manual
elseif u>=0.5
    y = 2;  % Semi-autonomous
else
    y = 1;  % Stabilized
end
